simulink model "BlokSchema"  (R2023b)
settings: Solver=VariableStepAuto  StartTime=0.0  StopTime=10000  RelTol=1e-3
values from neighbouring files (symbols this model uses):
  citatel = (K/(T1*T2))    (= 0.00186096256684)    [Zadanie2.m]
  Delay = 300    [Zadanie2.m]
  Grz_spatnaObdlMet = filt([q0 q1 q2], [1 -1], T)    [Zadanie2.m]
  Grz_tustin = c2d(Greg, T, 'tustin')    [Zadanie2.m]
  menovatel = [1,(T1+T2)/(T1*T2), 1/(T1*T2)]    [Zadanie2.m]
  T = 300    [Zadanie2.m]
settings Model: PacingRate=100  Creator=domin  LastModifiedBy=domin

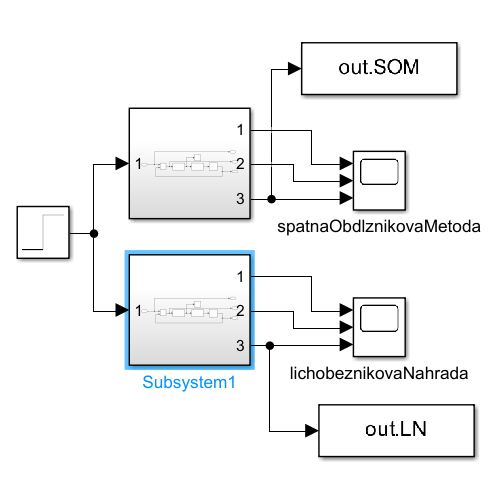
[thumbnail: Simulink's stored preview of the top-level diagram]
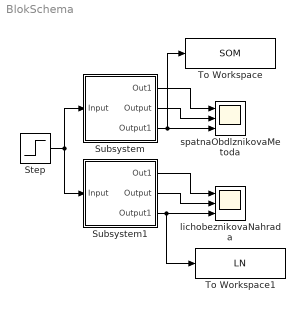
== system BlokSchema ==
  Step : Step  Time=0  Before=1  SampleTime=0
  Subsystem : Subsystem
  Subsystem1 : Subsystem
  To Workspace : ToWorkspace  VariableName=SOM  SampleTime=-1
  To Workspace1 : ToWorkspace  VariableName=LN  SampleTime=-1
  lichobeznikovaNahrada : Scope  NumInputPorts=3
  spatnaObdlznikovaMetoda : Scope  NumInputPorts=3
  wires:
  Step/1 -> Subsystem/1(Input), Subsystem1/1(Input)
  Subsystem/1(Out1) -> spatnaObdlznikovaMetoda/1
  Subsystem/2(Output) -> spatnaObdlznikovaMetoda/2
  Subsystem/3(Output1) -> To Workspace/1, spatnaObdlznikovaMetoda/3
  Subsystem1/1(Out1) -> lichobeznikovaNahrada/1
  Subsystem1/2(Output) -> lichobeznikovaNahrada/2
  Subsystem1/3(Output1) -> To Workspace1/1, lichobeznikovaNahrada/3

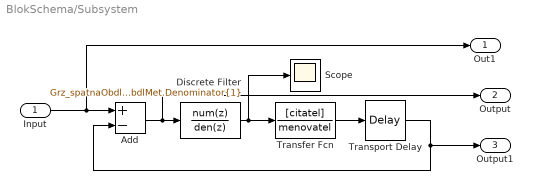
== system BlokSchema/Subsystem ==
  Input : Inport
  Add : Sum  Inputs=+-
  Discrete Filter : DiscreteFilter  Numerator=Grz_spatnaObdlMet.Numerator{1}  Denominator=Grz_spatnaObdlMet.Denominator{1}  SampleTime=T
  Scope : Scope
  Transfer Fcn : TransferFcn  Numerator=[citatel]  Denominator=menovatel
  Transport Delay : TransportDelay  DelayTime=Delay
  Out1 : Outport
  Output : Outport  Port=2
  Output1 : Outport  Port=3
  wires:
  Add/1 -> Discrete Filter/1, Output/1
  Input/1 -> Out1/1, Add/1
  Transfer Fcn/1 -> Transport Delay/1
  Discrete Filter/1 -> Transfer Fcn/1, Scope/1
  Transport Delay/1 -> Output1/1, Add/2

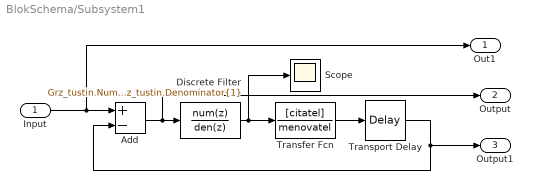
== system BlokSchema/Subsystem1 ==
  Input : Inport
  Add : Sum  Inputs=+-
  Discrete Filter : DiscreteFilter  Numerator=Grz_tustin.Numerator{1}  Denominator=Grz_tustin.Denominator{1}  SampleTime=T
  Scope : Scope
  Transfer Fcn : TransferFcn  Numerator=[citatel]  Denominator=menovatel
  Transport Delay : TransportDelay  DelayTime=Delay
  Out1 : Outport
  Output : Outport  Port=2
  Output1 : Outport  Port=3
  wires:
  Add/1 -> Discrete Filter/1, Output/1
  Input/1 -> Out1/1, Add/1
  Transfer Fcn/1 -> Transport Delay/1
  Discrete Filter/1 -> Transfer Fcn/1, Scope/1
  Transport Delay/1 -> Output1/1, Add/2
